simulink model "Save_Aligned_RGB_Depth_Videos"  (R2018b)
settings: Solver=FixedStepDiscrete  StartTime=0.0  StopTime=inf  FixedStep=0.001  RelTol=1e-3  EnableMultiTasking=on
undefined symbols (not defined in the file): datetime, Depth_, qc_get_step_size, RGB_, saved_data, Video3D
libraries: quarc_library x18
settings Model: SimulationMode=external  ExtModeTrigDuration=10000  Creator=glai  LastModifiedBy=glai
settings SolverCC: PositivePriorityOrder=on
settings HardwareCC: ProdBitPerLong=64  ProdHWDeviceType=Intel->x86-64 (Linux 64)
settings SFSimCC: SimUseLocalCustomCode=off
settings RTWCC: SystemTargetFile=quarc_linux_x64.tlc  TemplateMakefile=quarc_default_tmf  Description=QUARC Linux x64 Target (QDrone) Using Toolchain  RTWUseLocalCustomCode=off  Toolchain=QUARC linux_x64 | gmake (64-bit Windows)  BuildConfiguration=Faster Runs
settings CodeAppCC: StateflowObjectComments=on
settings STFCustomTargetCC: TargetLangStandard=C99 (ISO)  ConcurrentExecutionCompliant=on  GRTInterface=on  UseToolchainInfoCompliant=on  SystemTargetFile=quarc_linux_x64.tlc
settings GRTTargetCC: ParMdlRefBuildCompliant=off  CompOptLevelCompliant=off  CombineOutputUpdateFcns=off  MatFileLogging=off  CPPClassGenCompliant=off  GRTInterface=on  ExtMode=on  ExtModeMexFile=quarc_comm  ExtModeMexArgs='-w -d /tmp -uri %u','tcpip://192.168.2.X:17004'
settings ConfigComp: CovMetricSettings=dswe

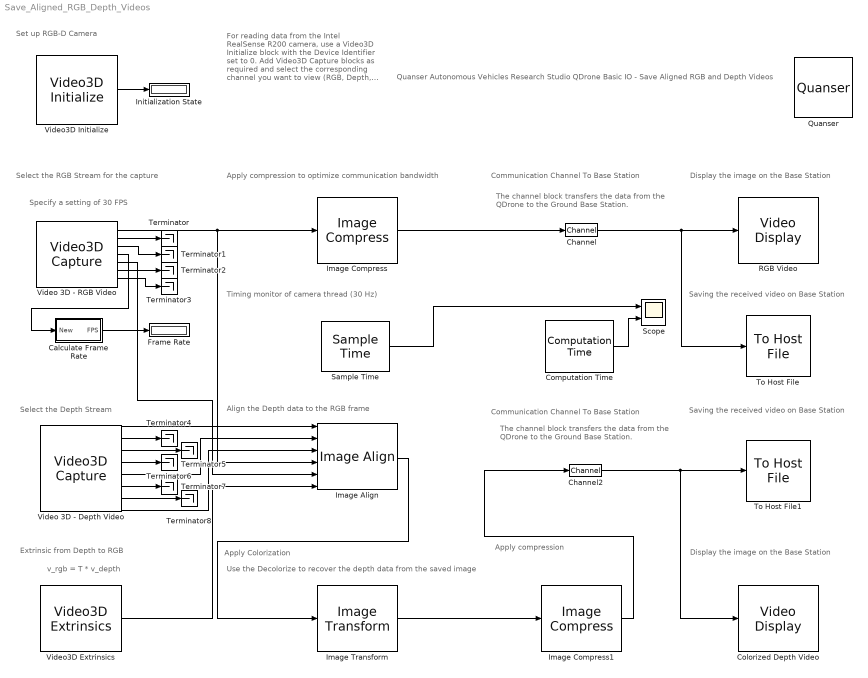
== system Save_Aligned_RGB_Depth_Videos ==
  note: Apply compression
  note: Use the Decolorize to recover the depth data from the saved image
  note: Apply Colorization
  note: Align the Depth data to the RGB frame
  note: v_rgb = T * v_depth
  note: Extrinsic from Depth to RGB
  note: Select the Depth Stream
  note: Saving the received video on Base Station
  note: Display the image on the Base Station
  note: The channel block transfers the data from the QDrone to the Ground Base Station.
  note: Communication Channel To Base Station
  note: Apply compression to optimize communication bandwidth
  note: Specify a setting of 30 FPS
  note: Select the RGB Stream for the capture
  note: Set up RGB-D Camera
  note: Quanser Autonomous Vehicles Research Studio
      | QDrone Basic IO - Save Aligned RGB and Depth Videos
  note: For reading data from the Intel RealSense R200 camera, use a Video3D Initialize block with the Device Identifier set to 0. Add Video3D Capture blocks as required and select the corresponding channel you want to view (RGB, Depth, Infrared, etc).
      |
      | Use a Video Compressed Display block to view the feed.
  note: Timing monitor of camera thread (30 Hz)
  note: The channel block transfers the data from the QDrone to the Ground Base Station.
  note: Communication Channel To Base Station
  note: Display the image on the Base Station
  note: Saving the received video on Base Station
  Calculate Frame Rate : Subsystem
  Channel : quarc_library/Signal Routing/Channel  channel=0  buffer_size=1
  Channel2 : quarc_library/Signal Routing/Channel  channel=1  buffer_size=1
  Colorized Depth Video : quarc_library/Multimedia/Video Display  Tag=Save_Aligned_RGB_Depth_Videos/Colorized Depth Video  sample_time=-1  use_hardware=on
  Computation Time : quarc_library/Sources/Time/Computation Time  sample_time=qc_get_step_size * ceil(1/30 / qc_get_step_size)  use_model=on  use_cpu_time=off
  Frame Rate : Display
      settings: Decimation=100
  Image Align : quarc_library/Image Processing/Generic/Image Align  direction=Depth to other
      settings: SourceProductName=QUARC Targets
  Image Compress : quarc_library/Image Processing/Generic/Image Compress  algorithm=JPEG  source=Internal dialog parameter  quality=50  output_dim=-1
  Image Compress1 : quarc_library/Image Processing/Generic/Image Compress  algorithm=JPEG  source=Internal dialog parameter  quality=50  output_dim=-1
  Image Transform : quarc_library/Image Processing/Generic/Image Transform  algorithm=Colorize  color_theme=KRYGCBMW  min_pixel=0  max_pixel=4000  focal_length=308  principal_point=[262 334]  radial_coeffs=[-0.3129 0.0907]  tangential_coeffs=[]  extrapolated_pixel=0  interpolation=nearest  row_coords=0  column_coords=0  output_height=480  output_width=640  angle=0  origin=[240 320]  output_origin=[240 320]  output_data_type=uint8
      settings: AttributesFormatString=(%<algorithm>)  SourceProductName=QUARC Targets
  Initialization State : Display
      settings: Decimation=100
  Quanser : quarc_library/Logos/Quanser
  RGB Video : quarc_library/Multimedia/Video Display  Tag=Save_Aligned_RGB_Depth_Videos/RGB Video  sample_time=-1  use_hardware=on
  Sample Time : quarc_library/Sources/Time/Sample Time  Priority=-99  sample_time=qc_get_step_size * ceil(1/30 / qc_get_step_size)
  Scope : Scope  NumInputPorts=2
  Terminator{,1..8} (9 alike) : Terminator
  To Host File : quarc_library/Sinks/To Host/To Host File  file_name=saved_data\RGB_%{char(datetime)}.mp4  variable_name=data  decimation=1  sample_time=-1  file_format=Video file  options=No header or footer  append=off  final_file_name=saved_data\RGB_2022-02-18 17-49-58.mp4  bitrate=2000000
  To Host File1 : quarc_library/Sinks/To Host/To Host File  file_name=saved_data\Depth_%{char(datetime)}.mp4  variable_name=data  decimation=1  sample_time=-1  file_format=Video file  options=No header or footer  append=off  final_file_name=saved_data\Depth_2022-02-18 17-49-58.mp4  bitrate=2000000
  Video 3D - Depth Video : quarc_library/Multimedia/Video3D Capture  object_name=Video3D-1  stream_type=Depth  stream_index=0  resolution=640 x 480  width=640  height=480  output_format=MATLAB greyscale (HxW)  data_type=uint16  sample_time=qc_get_step_size * ceil(1/30 / qc_get_step_size)  camera_intrinsics=on  depth_scale=on  brightness_override=off  brightness=50.0  contrast_override=off  contrast=50.0  hue_override=off  hue=50.0  saturation_override=off  saturation=50.0  sharpness_override=off  sharpness=50.0  gamma_override=off  gamma=50.0  gain_override=off  gain=50.0  backlightcompensation_override=off  backlightcompensation=50.0  whitebalance_override=Automatic white balance  whitebalance=50.0  exposure_override=Automatic exposure  exposure=30.0  emitter=Enable laser emitter  preset=Do not set camera presets
  Video 3D - RGB Video : quarc_library/Multimedia/Video3D Capture  object_name=Video3D-1  stream_type=RGB  stream_index=0  resolution=640 x 480  width=640  height=480  output_format=MATLAB RGB (HxWx3)  data_type=uint16  sample_time=qc_get_step_size * ceil(1/30 / qc_get_step_size)  camera_intrinsics=on  depth_scale=off  brightness_override=off  brightness=50.0  contrast_override=off  contrast=50.0  hue_override=off  hue=50.0  saturation_override=off  saturation=50.0  sharpness_override=off  sharpness=50.0  gamma_override=off  gamma=50.0  gain_override=off  gain=50.0  backlightcompensation_override=off  backlightcompensation=50.0  whitebalance_override=Automatic white balance  whitebalance=50.0  exposure_override=Automatic exposure  exposure=30.0  emitter=Enable laser emitter  preset=Do not set camera presets
  Video3D Extrinsics : quarc_library/Multimedia/Video3D Extrinsics  object_name=Video3D-1  from_block=Video 3D - Depth Video  to_block=Video 3D - RGB Video  sample_time=qc_get_step_size * ceil(1/30 / qc_get_step_size)
      settings: SourceProductName=QUARC Targets
  Video3D Initialize : quarc_library/Multimedia/Video3D Initialize  object_name=Video3D-1  source=Device  identifier=0  file=sample.bag  sample_time=qc_get_step_size * ceil(1/30 / qc_get_step_size)  active=on
  wires:
  Video3D Initialize/1 -> Initialization State/1
  Video 3D - RGB Video/4 -> Calculate Frame Rate/1(New)
  Calculate Frame Rate/1(FPS) -> Frame Rate/1
  Video 3D - RGB Video/2 -> Terminator/1
  Video 3D - RGB Video/3 -> Terminator1/1
  Video 3D - RGB Video/1 -> Image Align/4, Image Compress/1
  Image Compress/1 -> Channel/1
  Channel/1 -> RGB Video/1, To Host File/1
  Computation Time/1 -> Scope/2
  Sample Time/1 -> Scope/1
  Video 3D - RGB Video/6 -> Terminator2/1
  Video 3D - RGB Video/7 -> Terminator3/1
  Video 3D - Depth Video/1 -> Image Align/1
  Video 3D - Depth Video/8 -> Image Align/3
  Video 3D - Depth Video/5 -> Image Align/2
  Video 3D - RGB Video/5 -> Image Align/5
  Video3D Extrinsics/1 -> Image Align/6
  Image Align/1 -> Image Transform/1
  Channel2/1 -> Colorized Depth Video/1, To Host File1/1
  Video 3D - Depth Video/2 -> Terminator4/1
  Video 3D - Depth Video/3 -> Terminator5/1
  Video 3D - Depth Video/4 -> Terminator6/1
  Video 3D - Depth Video/6 -> Terminator7/1
  Video 3D - Depth Video/7 -> Terminator8/1
  Image Transform/1 -> Image Compress1/1
  Image Compress1/1 -> Channel2/1

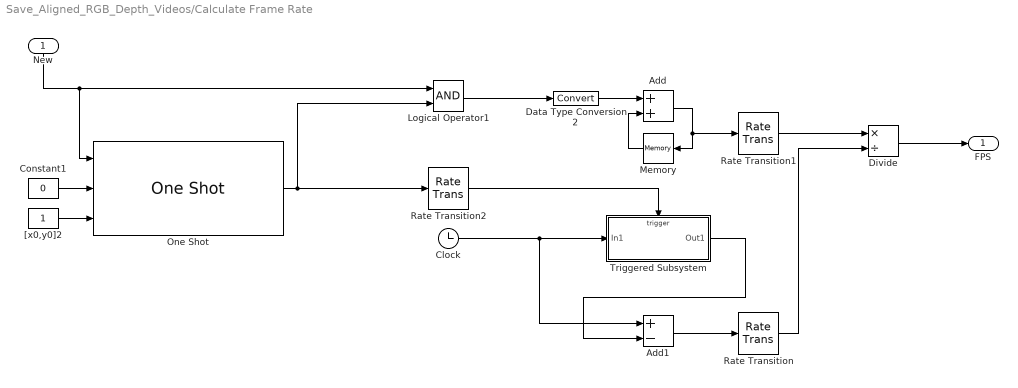
== system Save_Aligned_RGB_Depth_Videos/Calculate Frame Rate ==
  New : Inport
  Add : Sum
  Add1 : Sum  Inputs=+-
  Clock : Clock
  Constant1 : Constant  Value=0
  Data Type Conversion2 : DataTypeConversion
  Divide : Product  Inputs=*/
  Logical Operator1 : Logic  AllPortsSameDT=off  OutDataTypeStr=boolean
  Memory : Memory  InheritSampleTime=on
  One Shot : quarc_library/Discontinuities/One Shot  trigger_type=Rising edge  redun_pulse=Extend pulse width  width_source=Specify via dialog  pulse_width=1000
      settings: SourceProductName=QUARC Targets
  Rate Transition : RateTransition
  Rate Transition1 : RateTransition
  Rate Transition2 : RateTransition
  Triggered Subsystem : Subsystem  TreatAsAtomicUnit=on
  "[x0,y0]2" : Constant
  FPS : Outport
  wires:
  One Shot/1 -> Rate Transition2/1, Logical Operator1/2
  Add1/1 -> Rate Transition/1
  Rate Transition2/1 -> Triggered Subsystem/Trigger
  Data Type Conversion2/1 -> Add/1
  Logical Operator1/1 -> Data Type Conversion2/1
  "[x0,y0]2"/1 -> One Shot/3
  Constant1/1 -> One Shot/2
  New/1 -> One Shot/1, Logical Operator1/1
  Triggered Subsystem/1(Out1) -> Add1/2
  Rate Transition1/1 -> Divide/1
  Memory/1 -> Add/2
  Add/1 -> Memory/1, Rate Transition1/1
  Clock/1 -> Add1/1, Triggered Subsystem/1(In1)
  Rate Transition/1 -> Divide/2
  Divide/1 -> FPS/1

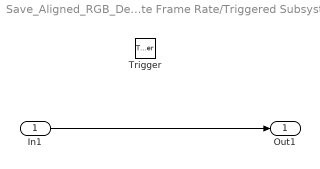
== system Save_Aligned_RGB_Depth_Videos/Calculate Frame Rate/Triggered Subsystem ==
  In1 : Inport
  Trigger : TriggerPort  VariantControl=Variant
  Out1 : Outport
  wires:
  In1/1 -> Out1/1
